simulink model "ct_system"  (R2022a)
settings: Solver=ode45  StartTime=0.0  StopTime=tfinal  FixedStep=T  MaxStep=0.01  RelTol=1e-12  AbsTol=1e-12  EnableMultiTasking=on
libraries: cstblocks x2
settings Model: Creator=cnielsen  LastModifiedBy=urban
settings SolverCC: AutoScaleAbsTol=off  AlgebraicLoopSolver=TrustRegion
settings DataIOCC: SaveFormat=Array  SignalLoggingSaveFormat=ModelDataLogs  SaveOutput=off  SaveTime=off  ReturnWorkspaceOutputs=off  Refine=5
settings OptimizationCC: ExpressionDepthLimit=2147483647  LifeSpan=inf
settings DebuggingCC: UnderspecifiedInitializationDetection=Classic  MergeDetectMultiDrivingBlocksExec=none  SolverPrmCheckMsg=warning  FcnCallInpInsideContextMsg=warning  UnconnectedInputMsg=warning  UnconnectedOutputMsg=warning  UnconnectedLineMsg=warning  StateNameClashWarn=warning  SFUnexpectedBacktrackingDiag=warning  SFNoUnconditionalDefaultTransitionDiag=warning  SFExecutionAtInitializationDiag=none  SFMachineParentedDataDiag=warning  ArithmeticOperatorsInVariantConditions=warning
settings HardwareCC: ProdBitPerPointer=32  ProdBitPerSizeT=32  ProdBitPerPtrDiffT=32  ProdLargestAtomicFloat=None  ProdIntDivRoundTo=Undefined  ProdEndianess=Unspecified  ProdWordSize=32  ProdHWDeviceType=32-bit Generic
settings ModelReferenceCC: PropagateSignalLabelsOutOfModel=off
settings SFSimCC: SimUseLocalCustomCode=off  CustomCodeUndefinedFunction=UseInterfaceOnly
settings RTWCC: RTWUseLocalCustomCode=off
settings CodeAppCC: StateflowObjectComments=on
settings GRTTargetCC: TargetLangStandard=C89/C90 (ANSI)  CombineOutputUpdateFcns=off  GRTInterface=on
settings ConfigComp: CovMetricSettings=dw  CovSaveCumulativeToWorkspaceVar=on  CovSaveSingleToWorkspaceVar=on  CovExternalEMLEnable=off

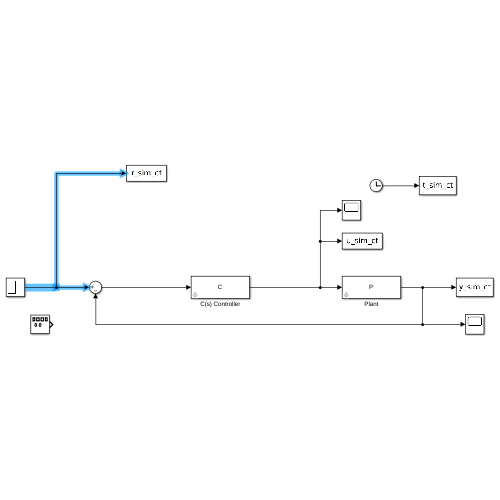
[thumbnail: Simulink's stored preview of the top-level diagram]
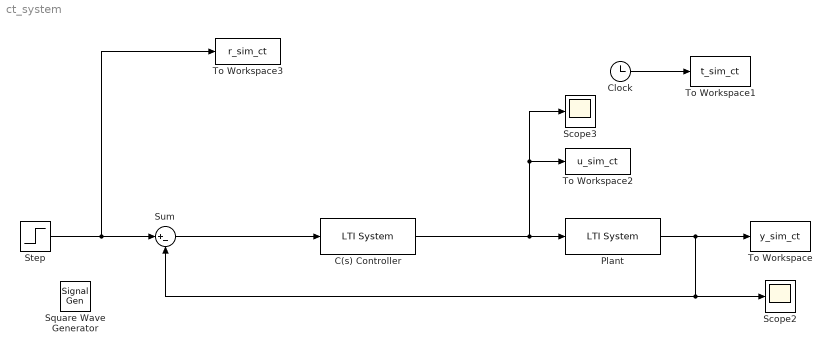
== system ct_system ==
  C(s) Controller : cstblocks/LTI System  sys=C  IC=[]
  Clock : Clock
  Plant : cstblocks/LTI System  sys=P  IC=[]
  Scope2 : Scope
  Scope3 : Scope
  Square Wave Generator : SignalGenerator  WaveForm=square  Units=rad/sec
  Step : Step  Time=0
  Sum : Sum  Inputs=|+-
  To Workspace : ToWorkspace  VariableName=y_sim_ct  SampleTime=-1
  To Workspace1 : ToWorkspace  VariableName=t_sim_ct  SampleTime=-1
  To Workspace2 : ToWorkspace  VariableName=u_sim_ct
  To Workspace3 : ToWorkspace  VariableName=r_sim_ct
  wires:
  Clock/1 -> To Workspace1/1
  Plant/1 -> To Workspace/1, Sum/2, Scope2/1
  C(s) Controller/1 -> Plant/1, To Workspace2/1, Scope3/1
  Sum/1 -> C(s) Controller/1
  Step/1 -> To Workspace3/1, Sum/1
